simulink model "FCElectricPlant"  (R2025b)
settings: Solver=VariableStepAuto  StartTime=0.0  StopTime=2474  RelTol=1e-3
model workspace (MAT data in the model file):
  Bat : object (value not decoded)
  BattDCDC : object (value not decoded)
  Brk : object (value not decoded)
  Cond : object (value not decoded)
  Cpl : object (value not decoded)
  DH2 = 74
  DH2O = 25
  DO2 = 18
  DRVctrl : object (value not decoded)
  Diff : object (value not decoded)
  Driveshaft : inertia (value not decoded)
  Duct : object (value not decoded)
  ElecThermal : object (value not decoded)
  FCDCDC : object (value not decoded)
  FCctrl : object (value not decoded)
  FTP72 : object (value not decoded)
  FTP75 : object (value not decoded)
  FinArea = 2
  FinDensity = 4
  H2_D = 74
  H2_R = 4124.48151676
  H2_T = [-56.55 -50 -40 -30 -20 -10 -5 -4 -3 -2 -1 0 ... (52 elements, 1x52)]
  H2_h = [2783.66044046 2873.94181646 3012.62601981 3152.22537302 3292.62486344 3433.7213836 3504.50184296 3518.67512521 3532.85394544 3547.03822323 3561.22787913 3575.42283463 ... (52 elements, 1x52)]
  H2_k = [142.834673487 146.602208511 152.236222043 157.732550942 163.09765294 168.338595937 170.914793442 171.426608923 171.937300227 172.446874689 172.955339635 173.462702375 ... (52 elements, 1x52)]
  H2_mu = [7.13280985169 7.28192581803 7.50683010986 7.72860158312 7.94743907375 8.16352107178 8.27057966039 8.29191522386 8.31322574339 8.33451136221 8.35577222214 8.37700846366 ... (52 elements, 1x52)]
  HWFET : object (value not decoded)
  Mot : object (value not decoded)
  N2_R = 296.802103844
  N2_T = [-56.55 -50 -40 -30 -20 -10 -5 -4 -3 -2 -1 0 ... (52 elements, 1x52)]
  N2_h = [224.312019476 231.141016529 241.564116975 251.984329606 262.402210767 272.818266127 278.025759131 279.06722248 280.10867517 281.150117667 282.191550441 283.232973957 ... (52 elements, 1x52)]
  N2_k = [19.6296532607 20.1533289725 20.9436243616 21.7231523445 22.4923063139 23.2514823267 23.6274403303 23.7023472872 23.7771601873 23.8518793809 23.9265052168 24.0010380424 ... (52 elements, 1x52)]
  N2_mu = [13.7948920665 14.1367187352 14.6513506072 15.1575394446 15.6556177861 16.1459023391 16.3882166949 16.4364580271 16.4846261831 16.532721447 16.5807441017 16.6286944287 ... (52 elements, 1x52)]
  NFin = 7680
  O2_D = 18
  O2_R = 259.836612623
  O2_T = [-56.55 -50 -40 -30 -20 -10 -5 -4 -3 -2 -1 0 ... (52 elements, 1x52)]
  O2_h = [196.314045635 202.302438243 211.445560194 220.590899229 229.740231593 238.895348953 243.475641264 244.39194743 245.308340402 246.224821996 247.14139403 248.05805832 ... (52 elements, 1x52)]
  O2_k = [19.6661951881 20.2224765128 21.0645207725 21.898029696 22.7232456338 23.5404090718 23.9460452976 24.0269406553 24.1077592592 24.1885013406 24.2691671302 24.349756858 ... (52 elements, 1x52)]
  O2_mu = [15.7665575307 16.1727626079 16.7849249434 17.3877315055 17.9815180942 18.5666055809 18.8559834763 18.9136105725 18.9711555252 19.0286186248 19.0860001607 19.1433004205 ... (52 elements, 1x52)]
  PTctrl : object (value not decoded)
  Pipe : object (value not decoded)
  Pump : object (value not decoded)
  RH2 = 4124.48291466
  RH2O = 461.523115726
  RH_a = 0.6
  RH_c = 0.6
  RN2 = 296.802204439
  RO2 = 259.836700689
  RelayVariant = 1
  ScenarioIndex = 5
  Sig : Simulink.Signal (value not decoded)
  SimEndTime = 2474
  T_cell = 80
  T_eff_bp = [0 20 40 60 80 100 120 140 160 180 200 220 ... (15 elements, 1x15)]
  T_env = 20
  T_ext = 30
  T_init = 303.15
  Tank : object (value not decoded)
  Tire : object (value not decoded)
  Tvec = [-50 -40 -30 -20 -10 0 10 20 30 40 50 60 ... (41 elements, 1x41)]
  US06 : object (value not decoded)
  UrbanCycle1 : object (value not decoded)
  UrbanCycle2 : object (value not decoded)
  UrbanCycle3 : object (value not decoded)
  UrbanCycle4 : object (value not decoded)
  UrbanCycle5 : object (value not decoded)
  Vehicle : object (value not decoded)
  WOT : object (value not decoded)
  anode_tube_D = 0.01
  cathode_tube_D = 0.05
  comp_mdot_corr_TLU = [0 0 0 0 0 0.2 0.15 0.1 0.05 0 0.4 0.3 ... (15 elements, 5x3)]
  comp_p_ratio_TLU = [1; 1.25; 1.5; 1.75; 2]
  comp_rpm_TLU = [0 1800 3600]
  coolant_num_layers = 20
  coolant_num_passes = 12
  coolant_tube_D = 0.05
  coolant_w_channels = 1
  drive_cycle_power = [0 0 0 0 0 0 0 0 0 0 0 0 ... (1050 elements, 1050x1)]
  drive_cycle_time = [0 3.15544362088e-30 0.0046730644306 0.0046730644306 0.0229169980413 0.0229169980413 0.0411609316521 0.0594048652628 0.0958927324843 0.168868466927 0.308339923682 0.308339923682 ... (1050 elements, 1050x1)]
  efficiency_table = [85 85 85 85 85 85 85 85 85 85 85 85 ... (180 elements, 12x15)]
  env_RH = 0.5
  env_T = 20
  env_p = 0.101325
  env_yO2 = 0.21
  f_fc_auxpower = [551.873653203 546.0853282 528.48462663 513.173595038 503.302975177 502.753456089 515.021163214 542.265022773 584.751680012 640.816461254 707.312051903 780.384247238 ... (869 elements, 79x11)]
  f_fc_currcmd_bpt = [0.209765 5.20060185897 10.1914387179 15.1822755769 20.1731124359 25.1639492949 30.1547861538 35.1456230128 40.1364598718 45.1272967308 50.1181335897 55.1089704487 ... (79 elements, 1x79)]
  f_fc_h2flow = [8.71593619412e-08 2.11208831613e-05 4.21802637945e-05 6.3315607286e-05 8.44733435522e-05 0.000105614873893 0.000126714989157 0.000147760022647 0.000168745833381 0.000189675717181 0.000210558338983 0.000231405772833 ... (869 elements, 79x11)]
  f_fc_heatflow = [-113.508553924 315.682858012 683.83093304 1077.33211881 1492.74924564 1928.28255982 2383.1090309 2856.86201514 3349.28475785 3860.05320307 4388.73420272 4934.82889994 ... (869 elements, 79x11)]
  f_fc_tmpcmd_bpt = [50 55 60 65 70 75 80 85 90 95 100]
  f_fc_voltage = [454.992615106 449.926167951 444.44198715 439.413829244 434.829610174 430.668984057 426.90491616 423.505302786 420.434569606 417.655187333 415.129053553 412.818701247 ... (869 elements, 79x11)]
  hH2 = [2873941.81645 3012626.01981 3152225.37301 3292624.86344 3433721.38359 3575422.83463 3717647.2553 3860321.98734 4003382.88163 4146773.54613 4290444.63593 4434353.18483 ... (41 elements, 1x41)]
  hH2O = [2407979.18389 2426599.35505 2445219.52621 2463839.69737 2482459.86853 2501080.03969 2520041.36444 2538661.5356 2557304.93352 2575974.09714 2594671.5511 2613399.77792 ... (41 elements, 1x41)]
  hN2 = [231141.016491 241564.116943 251984.329578 262402.210743 272818.266107 283232.973942 293646.803464 304060.22922 314473.742203 324887.858166 335303.123505 345720.119022 ... (41 elements, 1x41)]
  hO2 = [202302.438244 211445.560195 220590.89923 229740.231594 238895.348953 248058.05832 257230.174606 266413.508634 275609.852766 284820.965752 294048.557919 303294.277514 ... (41 elements, 1x41)]
  hvH2O = [2837864.0802 2838666.81899 2838713.54467 2838009.25742 2836579.406 2834477.18894 2477187.06302 2453519.25942 2429811.22988 2405977.28679 2381947.12654 2357654.5203 ... (41 elements, 1x41)]
  kH2 = [0.14660211438 0.15223611697 0.157732436203 0.163097529696 0.168338465237 0.173462565161 0.178477161614 0.183389433463 0.188206302164 0.192934369439 0.197579884152 0.202148729169 ... (41 elements, 1x41)]
  kH2O = [0.0133993325489 0.0140727292017 0.0147461258545 0.0154195225073 0.0160929191601 0.0167663158129 0.017416450238 0.0180898468908 0.0187835182831 0.019496836926 0.0202291830642 0.0209799564979 ... (41 elements, 1x41)]
  kN2 = [0.0201533289599 0.0209436243479 0.0217231523299 0.0224923062983 0.0232514823103 0.0240010380251 0.0247413260421 0.0254726839711 0.026195434744 0.0269098870397 0.0276163357829 0.028315062687 ... (41 elements, 1x41)]
  kO2 = [0.0202224764979 0.0210645207571 0.0218980296803 0.0227232456176 0.0235404090551 0.0243497568408 0.0251515209302 0.0259459275017 0.0267331962527 0.0275135401488 0.0282871691008 0.0290542796888 ... (41 elements, 1x41)]
  muH2 = [7.28192631884e-06 7.50683062629e-06 7.72860211493e-06 7.94743962074e-06 8.16352163375e-06 8.37700904042e-06 8.58804741514e-06 8.79676894741e-06 9.00329407235e-06 9.20773285791e-06 9.41018619135e-06 9.61074679906e-06 ... (41 elements, 1x41)]
  muH2O = [7.40754821278e-06 7.71570492949e-06 8.0238616462e-06 8.33201836291e-06 8.64017507962e-06 8.94833179633e-06 9.24231634895e-06 9.55047306566e-06 9.87031914628e-06 1.02003383346e-05 1.05392900589e-05 1.08861429187e-05 ... (41 elements, 1x41)]
  muN2 = [1.41367187228e-05 1.46513505944e-05 1.51575394313e-05 1.56556177724e-05 1.6145902325e-05 1.66286944141e-05 1.71042805521e-05 1.75729330776e-05 1.80349108304e-05 1.84904598363e-05 1.89398139868e-05 1.9383195703e-05 ... (41 elements, 1x41)]
  muO2 = [1.6172762594e-05 1.67849249289e-05 1.73877314906e-05 1.79815180788e-05 1.8566605565e-05 1.9143300404e-05 1.97118951916e-05 2.02726692488e-05 2.08258892185e-05 2.13718096611e-05 2.19106736419e-05 2.24427133044e-05 ... (41 elements, 1x41)]
  pH2O = [0.0039376926592 0.0128411282011 0.0380050105363 0.103238678713 0.259872929049 0.611151401419 1.22819893069 2.33931818334 4.24697083683 7.38493807375 12.3519458375 19.9464343078 ... (41 elements, 1x41)]
  p_a = 0.101325
  p_c = 0.101325
  p_sat = 0.0474144740302
  p_sat_c = 0.0474144740302
  p_sat_e = 0.00233931818334
  radiator_H = 0.5
  radiator_L = 1
  radiator_N_fins = 12000
  radiator_N_tubes = 25
  radiator_W = 0.025
  radiator_air_area_fins = 11.5625
  radiator_air_area_primary = 1.223125
  radiator_cp = 910
  radiator_eta_fin = 0.7
  radiator_fin_spacing = 0.002
  radiator_gap_H = 0.0192708333333
  radiator_rho = 2700
  radiator_t_wall = 0.0001
  radiator_tube_H = 0.0015
  radiator_tube_Leq = 2.5
  stack_D_gdl = 0.07
  stack_alpha = 0.6
  stack_area = 280
  stack_iL = 1.4
  stack_io = 0.0001
  stack_mea_cp = 870
  stack_mea_rho = 1800
  stack_membrane_MW = 1.1
  stack_membrane_rho = 2000
  stack_num_cells = 400
  stack_num_channels = 8
  stack_t_gdl = 250
  stack_t_membrane = 125
  stack_w_channels = 1
  tank_V = 120
  tank_p = 70
  tank_yH2 = 0.9997
  y_H2O_a = 0.280766685597
  y_H2O_c = 0.0138523652603
  y_H2_a = 0.719233314403
  y_N2_a = 0
  y_N2_c = 0.77614763474
  y_O2_c = 0.21
symbols that are objects in the model workspace (value not decoded): Bat, ElecThermal, Mot
libraries: fl_lib x91, nesl_utility x43, autolibpowerinfoutils x9, SimscapeFluids_lib x5, ee_lib x3, slpidlib x2, batteryecm_lib x1, simulink_extras x1, simulink x1
(part 4 of 4)

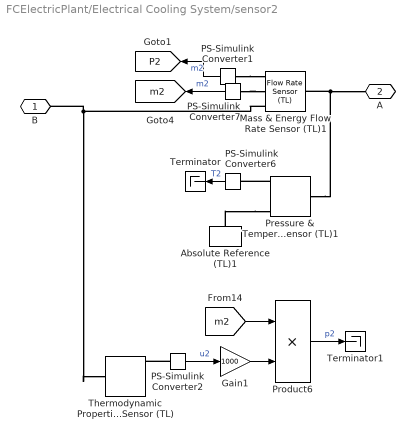
== system FCElectricPlant/Electrical Cooling System/sensor2 ==
  Absolute Reference (TL)1 : fl_lib/Thermal Liquid/Elements/Absolute Reference (TL)
  Gain1 : Gain  Gain=1000
  Mass & Energy Flow Rate Sensor (TL)1 : fl_lib/Thermal Liquid/Sensors/Flow Rate Sensor (TL)  mass_flow_measure=true  volumetric_flow_measure=false  energy_flow_measure=true
      settings: InternalSimscapePortConfiguration="{\"Bottom\":[{\"id\":\"PHI\",\"label\":\"φ\",\"type\":\"output\"}],\"Left\":[{\"id\":\"A\",\"label\":\"A\",\"type\":\"foundation.thermal_liquid.thermal_liquid\"}],\"Right\":[{\"id\":\"B\",\"label\":\"B\",\"type\":\"foundation.thermal_liquid.thermal_liquid\"},{\"id\":\"M\",\"label\":\"M\",\"type\":\"output\"}],\"Top\":[]}"
  PS-Simulink Converter{1..2,6..7} (4 alike) : nesl_utility/PS-Simulink Converter  PhysicalDomain=network_engine_domain  SubClassName=ps_output  LeftPortType=input  RightPortType=output  PseudoPeriodic=off  Frequencies=[]  VectorFormat=inherit  Unit=inherit  AffineConversion=off
  Pressure & Temperature Sensor (TL)1 : fl_lib/Thermal Liquid/Sensors/Pressure & Temperature Sensor (TL)  reference=foundation.enum.MeasurementReference.difference  pressure=true  pressure_spec=foundation.enum.PressureMeasementSpec.Absolute  temperature=true
      settings: InternalSimscapePortConfiguration="{\"Bottom\":[{\"id\":\"T\",\"label\":\"T\",\"type\":\"output\"}],\"Left\":[{\"id\":\"A\",\"label\":\"A\",\"type\":\"foundation.thermal_liquid.thermal_liquid\"}],\"Right\":[{\"id\":\"B\",\"label\":\"B\",\"type\":\"foundation.thermal_liquid.thermal_liquid\"},{\"id\":\"P\",\"label\":\"P\",\"type\":\"output\"}],\"Top\":[]}"
  Product6 : Product
  Terminator : Terminator
  Terminator1 : Terminator
  Thermodynamic Properties Sensor (TL) : fl_lib/Thermal Liquid/Sensors/Thermodynamic Properties Sensor (TL)  internal_energy=true  density=true  specific_heat=true
      settings: InternalSimscapePortConfiguration="{\"Bottom\":[],\"Left\":[{\"id\":\"A\",\"label\":\"A\",\"type\":\"foundation.thermal_liquid.thermal_liquid\"}],\"Right\":[{\"id\":\"U\",\"label\":\"u\",\"type\":\"output\"},{\"id\":\"RHO\",\"label\":\"ρ\",\"type\":\"output\"},{\"id\":\"CP\",\"label\":\"cp\",\"type\":\"output\"}],\"Top\":[]}"
  B : PMIOPort  Side=Left
  A : PMIOPort  Port=2  Side=Right
  tag scope: P2=global, m2=global
  wires:
  PS-Simulink Converter6/1 -> Terminator/1  "T2"
  PS-Simulink Converter7/1 -> [m2]  "m2"
  Product6/1 -> Terminator1/1  "p2"
  Gain1/1 -> Product6/2
  PS-Simulink Converter2/1 -> Gain1/1  "u2"
  [m2] -> Product6/1
  PS-Simulink Converter1/1 -> [P2]  "m2"
  connections:
  Pressure & Temperature Sensor (TL)1/LConn1 -- A/RConn1 -- Mass & Energy Flow Rate Sensor (TL)1/LConn1
  PS-Simulink Converter7/LConn1 -- Mass & Energy Flow Rate Sensor (TL)1/RConn2
  Mass & Energy Flow Rate Sensor (TL)1/RConn1 -- Thermodynamic Properties Sensor (TL)/LConn1 -- B/RConn1
  Pressure & Temperature Sensor (TL)1/RConn3 -- PS-Simulink Converter6/LConn1
  PS-Simulink Converter2/LConn1 -- Thermodynamic Properties Sensor (TL)/RConn1
  Absolute Reference (TL)1/LConn1 -- Pressure & Temperature Sensor (TL)1/RConn1
  PS-Simulink Converter1/LConn1 -- Mass & Energy Flow Rate Sensor (TL)1/RConn3

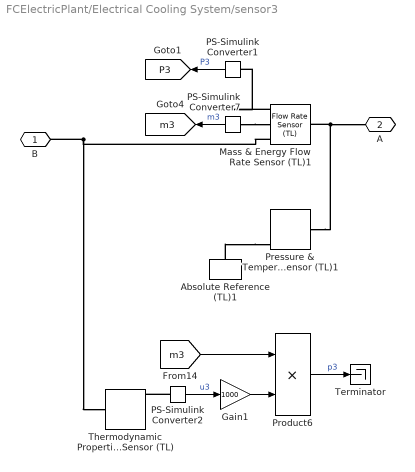
== system FCElectricPlant/Electrical Cooling System/sensor3 ==
  Absolute Reference (TL)1 : fl_lib/Thermal Liquid/Elements/Absolute Reference (TL)
  Gain1 : Gain  Gain=1000
  Mass & Energy Flow Rate Sensor (TL)1 : fl_lib/Thermal Liquid/Sensors/Flow Rate Sensor (TL)  mass_flow_measure=true  volumetric_flow_measure=false  energy_flow_measure=true
      settings: InternalSimscapePortConfiguration="{\"Bottom\":[{\"id\":\"PHI\",\"label\":\"φ\",\"type\":\"output\"}],\"Left\":[{\"id\":\"A\",\"label\":\"A\",\"type\":\"foundation.thermal_liquid.thermal_liquid\"}],\"Right\":[{\"id\":\"B\",\"label\":\"B\",\"type\":\"foundation.thermal_liquid.thermal_liquid\"},{\"id\":\"M\",\"label\":\"M\",\"type\":\"output\"}],\"Top\":[]}"
  PS-Simulink Converter1 : nesl_utility/PS-Simulink Converter  PhysicalDomain=network_engine_domain  SubClassName=ps_output  LeftPortType=input  RightPortType=output  PseudoPeriodic=off  Frequencies=[]  VectorFormat=inherit  Unit=inherit  AffineConversion=off
  PS-Simulink Converter2 : nesl_utility/PS-Simulink Converter  PhysicalDomain=network_engine_domain  SubClassName=ps_output  LeftPortType=input  RightPortType=output  PseudoPeriodic=off  Frequencies=[]  VectorFormat=inherit  Unit=inherit  AffineConversion=off
  PS-Simulink Converter7 : nesl_utility/PS-Simulink Converter  PhysicalDomain=network_engine_domain  SubClassName=ps_output  LeftPortType=input  RightPortType=output  PseudoPeriodic=off  Frequencies=[]  VectorFormat=inherit  Unit=inherit  AffineConversion=off
  Pressure & Temperature Sensor (TL)1 : fl_lib/Thermal Liquid/Sensors/Pressure & Temperature Sensor (TL)  reference=foundation.enum.MeasurementReference.difference  pressure=true  pressure_spec=foundation.enum.PressureMeasementSpec.Absolute  temperature=true
      settings: InternalSimscapePortConfiguration="{\"Bottom\":[{\"id\":\"T\",\"label\":\"T\",\"type\":\"output\"}],\"Left\":[{\"id\":\"A\",\"label\":\"A\",\"type\":\"foundation.thermal_liquid.thermal_liquid\"}],\"Right\":[{\"id\":\"B\",\"label\":\"B\",\"type\":\"foundation.thermal_liquid.thermal_liquid\"},{\"id\":\"P\",\"label\":\"P\",\"type\":\"output\"}],\"Top\":[]}"
  Product6 : Product
  Terminator : Terminator
  Thermodynamic Properties Sensor (TL) : fl_lib/Thermal Liquid/Sensors/Thermodynamic Properties Sensor (TL)  internal_energy=true  density=true  specific_heat=true
      settings: InternalSimscapePortConfiguration="{\"Bottom\":[],\"Left\":[{\"id\":\"A\",\"label\":\"A\",\"type\":\"foundation.thermal_liquid.thermal_liquid\"}],\"Right\":[{\"id\":\"U\",\"label\":\"u\",\"type\":\"output\"},{\"id\":\"RHO\",\"label\":\"ρ\",\"type\":\"output\"},{\"id\":\"CP\",\"label\":\"cp\",\"type\":\"output\"}],\"Top\":[]}"
  B : PMIOPort  Side=Left
  A : PMIOPort  Port=2  Side=Right
  tag scope: P3=global, m3=global
  wires:
  [m3] -> Product6/1
  PS-Simulink Converter2/1 -> Gain1/1  "u3"
  Gain1/1 -> Product6/2
  PS-Simulink Converter7/1 -> [m3]  "m3"
  PS-Simulink Converter1/1 -> [P3]  "P3"
  Product6/1 -> Terminator/1  "p3"
  connections:
  Absolute Reference (TL)1/LConn1 -- Pressure & Temperature Sensor (TL)1/RConn1
  PS-Simulink Converter2/LConn1 -- Thermodynamic Properties Sensor (TL)/RConn1
  B/RConn1 -- Thermodynamic Properties Sensor (TL)/LConn1 -- Mass & Energy Flow Rate Sensor (TL)1/RConn1
  PS-Simulink Converter7/LConn1 -- Mass & Energy Flow Rate Sensor (TL)1/RConn2
  Mass & Energy Flow Rate Sensor (TL)1/LConn1 -- A/RConn1 -- Pressure & Temperature Sensor (TL)1/LConn1
  Mass & Energy Flow Rate Sensor (TL)1/RConn3 -- PS-Simulink Converter1/LConn1

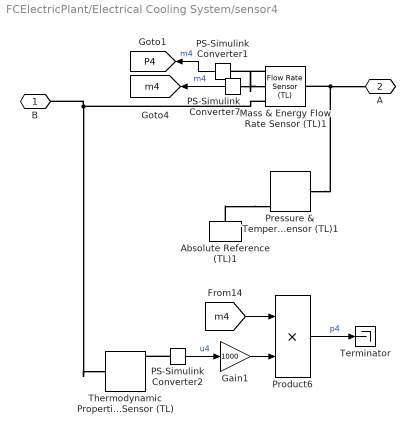
== system FCElectricPlant/Electrical Cooling System/sensor4 ==
  Absolute Reference (TL)1 : fl_lib/Thermal Liquid/Elements/Absolute Reference (TL)
  Gain1 : Gain  Gain=1000
  Mass & Energy Flow Rate Sensor (TL)1 : fl_lib/Thermal Liquid/Sensors/Flow Rate Sensor (TL)  mass_flow_measure=true  volumetric_flow_measure=false  energy_flow_measure=true
      settings: InternalSimscapePortConfiguration="{\"Bottom\":[{\"id\":\"PHI\",\"label\":\"φ\",\"type\":\"output\"}],\"Left\":[{\"id\":\"A\",\"label\":\"A\",\"type\":\"foundation.thermal_liquid.thermal_liquid\"}],\"Right\":[{\"id\":\"B\",\"label\":\"B\",\"type\":\"foundation.thermal_liquid.thermal_liquid\"},{\"id\":\"M\",\"label\":\"M\",\"type\":\"output\"}],\"Top\":[]}"
  PS-Simulink Converter1 : nesl_utility/PS-Simulink Converter  PhysicalDomain=network_engine_domain  SubClassName=ps_output  LeftPortType=input  RightPortType=output  PseudoPeriodic=off  Frequencies=[]  VectorFormat=inherit  Unit=inherit  AffineConversion=off
  PS-Simulink Converter2 : nesl_utility/PS-Simulink Converter  PhysicalDomain=network_engine_domain  SubClassName=ps_output  LeftPortType=input  RightPortType=output  PseudoPeriodic=off  Frequencies=[]  VectorFormat=inherit  Unit=inherit  AffineConversion=off
  PS-Simulink Converter7 : nesl_utility/PS-Simulink Converter  PhysicalDomain=network_engine_domain  SubClassName=ps_output  LeftPortType=input  RightPortType=output  PseudoPeriodic=off  Frequencies=[]  VectorFormat=inherit  Unit=inherit  AffineConversion=off
  Pressure & Temperature Sensor (TL)1 : fl_lib/Thermal Liquid/Sensors/Pressure & Temperature Sensor (TL)  reference=foundation.enum.MeasurementReference.difference  pressure=true  pressure_spec=foundation.enum.PressureMeasementSpec.Absolute  temperature=true
      settings: InternalSimscapePortConfiguration="{\"Bottom\":[{\"id\":\"T\",\"label\":\"T\",\"type\":\"output\"}],\"Left\":[{\"id\":\"A\",\"label\":\"A\",\"type\":\"foundation.thermal_liquid.thermal_liquid\"}],\"Right\":[{\"id\":\"B\",\"label\":\"B\",\"type\":\"foundation.thermal_liquid.thermal_liquid\"},{\"id\":\"P\",\"label\":\"P\",\"type\":\"output\"}],\"Top\":[]}"
  Product6 : Product
  Terminator : Terminator
  Thermodynamic Properties Sensor (TL) : fl_lib/Thermal Liquid/Sensors/Thermodynamic Properties Sensor (TL)  internal_energy=true  density=true  specific_heat=true
      settings: InternalSimscapePortConfiguration="{\"Bottom\":[],\"Left\":[{\"id\":\"A\",\"label\":\"A\",\"type\":\"foundation.thermal_liquid.thermal_liquid\"}],\"Right\":[{\"id\":\"U\",\"label\":\"u\",\"type\":\"output\"},{\"id\":\"RHO\",\"label\":\"ρ\",\"type\":\"output\"},{\"id\":\"CP\",\"label\":\"cp\",\"type\":\"output\"}],\"Top\":[]}"
  B : PMIOPort  Side=Left
  A : PMIOPort  Port=2  Side=Right
  tag scope: P4=global, m4=global
  wires:
  PS-Simulink Converter7/1 -> [m4]  "m4"
  Product6/1 -> Terminator/1  "p4"
  Gain1/1 -> Product6/2
  PS-Simulink Converter2/1 -> Gain1/1  "u4"
  [m4] -> Product6/1
  PS-Simulink Converter1/1 -> [P4]  "m4"
  connections:
  Pressure & Temperature Sensor (TL)1/LConn1 -- A/RConn1 -- Mass & Energy Flow Rate Sensor (TL)1/LConn1
  PS-Simulink Converter7/LConn1 -- Mass & Energy Flow Rate Sensor (TL)1/RConn2
  Mass & Energy Flow Rate Sensor (TL)1/RConn1 -- Thermodynamic Properties Sensor (TL)/LConn1 -- B/RConn1
  PS-Simulink Converter2/LConn1 -- Thermodynamic Properties Sensor (TL)/RConn1
  Absolute Reference (TL)1/LConn1 -- Pressure & Temperature Sensor (TL)1/RConn1
  Mass & Energy Flow Rate Sensor (TL)1/RConn3 -- PS-Simulink Converter1/LConn1

== system FCElectricPlant/Fuel Cell/Converter Control ==
  FCCurrCmd : Inport
  FCCurr : Inport  Port=2
  Add : Sum
  Add1 : Sum  Inputs=-+
  Compare To Constant : simulink/Logic and Bit Operations/Compare To Constant  relop=<=  const=0.01  OutDataTypeStr=boolean  ZeroCross=off
  Constant : Constant  Value=0
  Constant3 : Constant  Value=0
  PID Controller : slpidlib/PID Controller  Controller=PID  Form=Parallel  TimeDomain=Continuous-time  UseExternalTs=off  SampleTime=-1  IntegratorMethod=Forward Euler  FilterMethod=Forward Euler  ControllerParametersSource=internal  P=0.006  I=0.01  UseKiTs=off  D=0  UseExternalDerivativeSource=off  N=100  UseFilter=on  TunerSelectOption=Transfer Function Based (PID Tuner App)  InitialConditionSource=external  InitialConditionForIntegrator=0  InitialConditionForFilter=0  DifferentiatorICPrevScaledInput=0  ExternalReset=falling  TrackingMode=off  Kt=1  LimitOutput=on  SatLimitsSource=internal  UpperSaturationLimit=1  LowerSaturationLimit=-1  LinearizeAsGain=on  AntiWindupMode=none  Kb=1  LimitIntegrator=off  UpperIntegratorSaturationLimit=inf  LowerIntegratorSaturationLimit=-inf  POutMin=[]  POutMax=[]  IOutMin=[]  IOutMax=[]  DOutMin=[]  DOutMax=[]  NOutMin=[]  NOutMax=[]  SumOutMin=[]  SumOutMax=[]  SaturationOutMin=[]  SaturationOutMax=[]  PParamMin=[]  PParamMax=[]  IParamMin=[]  IParamMax=[]  DParamMin=[]  DParamMax=[]  NParamMin=[]  NParamMax=[]  KbParamMin=[]  KbParamMax=[]  KtParamMin=[]  KtParamMax=[]  KbOutMin=[]  KbOutMax=[]  KtOutMin=[]  KtOutMax=[]  IntegratorOutMin=[]  IntegratorOutMax=[]  FilterOutMin=[]  FilterOutMax=[]  SumI1OutMin=[]  SumI1OutMax=[]  SumI2OutMin=[]  SumI2OutMax=[]  SumI3OutMin=[]  SumI3OutMax=[]  SumI4OutMin=[]  SumI4OutMax=[]  SumDOutMin=[]  SumDOutMax=[]  DifferentiatorOutMin=[]  DifferentiatorOutMax=[]  FilterDiffOutCoefMin=[]  FilterDiffOutCoefMax=[]  ReciprocalOutMin=[]  ReciprocalOutMax=[]  SumDenOutMin=[]  SumDenOutMax=[]  SumNumOutMin=[]  SumNumOutMax=[]  DivideOutMin=[]  DivideOutMax=[]  UdiffTsProdOutMin=[]  UdiffTsProdOutMax=[]  NTsProdOutMin=[]  NTsProdOutMax=[]  UintegralTsProdOutMin=[]  UintegralTsProdOutMax=[]  UngainTsProdOutMin=[]  UngainTsProdOutMax=[]  ClampingZeroOutDataTypeStr=Inherit: Inherit via back propagation  ClampingZeroOutMin=[]  ClampingZeroOutMax=[]  FilterDenConstantOutDataTypeStr=Inherit: Inherit via back propagation  FilterDenConstantOutMin=[]  FilterDenConstantOutMax=[]  PCopyOutDataTypeStr=Inherit: Inherit via back propagation  PCopyOutMin=[]  PCopyOutMax=[]  NCopyOutDataTypeStr=Inherit: Inherit via back propagation  NCopyOutMin=[]  NCopyOutMax=[]  IntegratorContinuousStateAttributes=''  IntegratorStateMustResolveToSignalObject=off  IntegratorRTWStateStorageClass=Auto  FilterContinuousStateAttributes=''  FilterStateMustResolveToSignalObject=off  FilterRTWStateStorageClass=Auto  ParallelPVariant=InternalParameters  IdealPVariant=Disabled  IVariant=InternalParameters  DVariant=InternalParameters  IntegratorVariant=Continuous  SatVariant=Enabled  AWVariant=Passthrough  PCopyVariant=Disabled  TRVariant=Disabled  FdbkBlocksVariant=Forward  IdealPFdbkVariant=Disabled  SatFdbkVariant=Disabled  DerivativeFilterVariant=ContFilter  NVariant=InternalParameters  NCopyVariant=Disabled  FilterICVariant=ExternalICs  IntegratorICVariant=ExternalICs  ExternalResetVariant=ExternalReset  TRSumVariant=Passthrough  SumFdbkVariant=Disabled  SumVariant=Sum_PID  TsampFilterVariant=InternalTs  TsampNgainVariant=Passthrough  TsampIntegralVariant=Disabled_SignalSpec  ExternalSaturationOutDataTypeStr=Inherit: Same as second input  DerivativeSourceVariant=ErrorSignal  PreIntVariant=InternalPreInt
  Saturation : Saturate  UpperLimit=1  LowerLimit=0  ZeroCross=off
  Transfer Fcn : TransferFcn  Denominator=[0.001 1]
  u_boost : Outport
  wires:
  Constant3/1 -> Add/2
  PID Controller/1 -> Add/1, Transfer Fcn/1
  FCCurr/1 -> Add1/1
  Add/1 -> Saturation/1
  FCCurrCmd/1 -> Compare To Constant/1, Add1/2
  Add1/1 -> PID Controller/1
  Transfer Fcn/1 -> PID Controller/3
  Constant/1 -> PID Controller/4
  Compare To Constant/1 -> PID Controller/2
  Saturation/1 -> u_boost/1

== system FCElectricPlant/Fuel Cell/Fuel Cell ==
  i_cmd : Inport
  FCTempCmd : Inport  Port=2
  Lookup Table Fuel Cell : Subsystem  VariantControl=LookupTableFuelCell
      settings: PortSchema="{\"entries\":[{\"content\":{\"sides\":[{\"content\":{\"connectorIds\":[]},\"type\":\"ConnectorPlacement.EquallySpacedRectSide\",\"uuid\":\"32248e1c-8adb-4301-a735-652c844f38d9\"},{\"content\":{\"connectorIds\":[],\"side\":\"RIGHT\"},\"type\":\"ConnectorPlacement.EquallySpacedRectSide\",\"uuid\":\"e199895e-2a46-4791-8ec6-c72fbddb281a\"},{\"content\":{\"connectorIds\":[\"In1\",\"In2\"],\"side\":\"TOP\"},\"type\":\"ConnectorPlacement.EquallySpacedRectSide\",\"uuid\":\"d27f5cfc-8d50-4a08-b63d-60966cdd3a3e\"},{\"content\":{\"connectorIds\":[\"Out1\",\"Out2\",\"Out3\",\"Out4\",\"RConn1\",\"RConn2\"],\"side\":\"BOTTOM\"},\"type\":\"ConnectorPlacement.EquallySpacedRectSide\",\"uuid\":\"4de9f516-5cfd-4c93-92a2-161937995774\"}]},\"type\":\"ConnectorPlacement.EquallySpacedConnector\",\"uuid\":\"ebb74780-6fd4-4e24-9636-290cc1e1e603\"}],\"packageUris\":[\"http://schema.mathworks.com/mf0/Connector/R2020b\"],\"version\":\"1.0\"}"
  Simscape Fuel Cell : Subsystem  VariantControl=SimscapeFuelCell  ReferencedSubsystem=SSCFuelCell
  + : PMIOPort  Side=Right
  - : PMIOPort  Port=2  Side=Right
  FCCurr : Outport
  FCVolt : Outport  Port=2
  Pt : Outport  Port=3
  H2Flow : Outport  Port=4

== system FCElectricPlant/Fuel Cell/Thermal1 ==
  Controlled Heat Flow Rate Source : fl_lib/Thermal/Thermal Sources/Controlled Heat Flow Rate Source
  PS Gain : fl_lib/Physical Signals/Functions/PS Gain  gain=0.001 Ohm
  PS Math Function : fl_lib/Physical Signals/Functions/PS Math Function  fcn_choice=foundation.enum.math_function.square  v=1
  Thermal Mass : fl_lib/Thermal/Thermal Elements/Thermal Mass  mass_type=foundation.enum.constant_variable.constant  mass=500 kg  sp_heat=447 J/kg/K  mass_min=1e-6 kg  num_ports=foundation.enum.numPorts2.one  m_specify=off  m_priority=High  m=1 kg  m_nominal_specify=off  m_nominal_value=1  m_nominal_unit=kg  T_specify=off  T_priority=High  T=300 K  T_nominal_specify=off  T_nominal_value=1  T_nominal_unit=K  Q_specify=off  Q_priority=None  Q=0 W  Q_nominal_specify=off  Q_nominal_value=1  Q_nominal_unit=W
  Thermal Reference2 : fl_lib/Thermal/Thermal Elements/Thermal Reference
  H : PMIOPort  Side=Right
  i : PMIOPort  Port=2  Side=Left
  connections:
  H/RConn1 -- Controlled Heat Flow Rate Source/LConn1 -- Thermal Mass/LConn1
  i/RConn1 -- PS Math Function/LConn1
  Thermal Reference2/LConn1 -- Controlled Heat Flow Rate Source/RConn2
  PS Math Function/RConn1 -- PS Gain/LConn1
  Controlled Heat Flow Rate Source/RConn1 -- PS Gain/RConn1

== system FCElectricPlant/Motor/Elec Sensor ==
  Current Sensor2 : fl_lib/Electrical/Electrical Sensors/Current Sensor
  Electrical Reference : fl_lib/Electrical/Electrical Elements/Electrical Reference
  PS-Simulink Converter : nesl_utility/PS-Simulink Converter  PhysicalDomain=network_engine_domain  SubClassName=ps_output  LeftPortType=input  RightPortType=output  PseudoPeriodic=off  Frequencies=[]  VectorFormat=1-D array  Unit=inherit  AffineConversion=off
  PS-Simulink Converter4 : nesl_utility/PS-Simulink Converter  PhysicalDomain=network_engine_domain  SubClassName=ps_output  LeftPortType=input  RightPortType=output  PseudoPeriodic=off  Frequencies=[]  VectorFormat=1-D array  Unit=1  AffineConversion=off
  Product2 : Product
  Terminator : Terminator
  Voltage Sensor : fl_lib/Electrical/Electrical Sensors/Voltage Sensor
  + : PMIOPort  Side=Left
  - : PMIOPort  Port=2  Side=Right
  wires:
  PS-Simulink Converter4/1 -> Product2/2  "MotCurr"
  Product2/1 -> Terminator/1  "MotPwrElec"
  PS-Simulink Converter/1 -> Product2/1  "MotV"
  connections:
  Current Sensor2/RConn1 -- PS-Simulink Converter4/LConn1
  Current Sensor2/RConn2 -- -/RConn1
  +/RConn1 -- Voltage Sensor/LConn1 -- Current Sensor2/LConn1
  Electrical Reference/LConn1 -- Voltage Sensor/RConn2
  PS-Simulink Converter/LConn1 -- Voltage Sensor/RConn1

== system FCElectricPlant/Motor/Simulink Interface ==
  MotSpd : Inport
  Ideal Angular Velocity Source1 : fl_lib/Mechanical/Mechanical Sources/Ideal Angular Velocity Source
  Ideal Torque Sensor1 : fl_lib/Mechanical/Mechanical Sensors/Ideal Torque Sensor
  Ideal Torque Sensor2 : fl_lib/Mechanical/Mechanical Sensors/Ideal Torque Sensor
  Motor Coupling Dynamics1 : TransferFcn  Denominator=[0.001 1]
  PS-Simulink Converter2 : nesl_utility/PS-Simulink Converter  PhysicalDomain=network_engine_domain  SubClassName=ps_output  LeftPortType=input  RightPortType=output  PseudoPeriodic=off  Frequencies=[]  VectorFormat=1-D array  Unit=1  AffineConversion=off
  Product1 : Product
  Simulink-PS Converter4 : nesl_utility/Simulink-PS Converter  PhysicalDomain=network_engine_domain  SubClassName=ps_input  LeftPortType=input  RightPortType=output  PseudoPeriodic=off  Frequencies=[]  NoiseDistribution=none  NoiseParameters=[]  Unit=rad/s  AffineConversion=off  FilteringAndDerivatives=filter  SimscapeFilterOrder=1  InputFilterTimeConstant=0.001  UdotUserProvided=0
  Terminator : Terminator
  Transfer Fcn2 : TransferFcn  Denominator=[0.001 1]
  C : PMIOPort  Side=Left
  R : PMIOPort  Port=2  Side=Left
  MotTrq : Outport
  wires:
  Motor Coupling Dynamics1/1 -> MotTrq/1  "MotTrq"
  MotSpd/1 -> Transfer Fcn2/1
  PS-Simulink Converter2/1 -> Product1/1, Motor Coupling Dynamics1/1
  Transfer Fcn2/1 -> Product1/2, Simulink-PS Converter4/1
  Product1/1 -> Terminator/1  "MotPwrMech"
  connections:
  Ideal Torque Sensor2/RConn2 -- PS-Simulink Converter2/LConn1
  Ideal Angular Velocity Source1/LConn1 -- Ideal Torque Sensor1/RConn1
  Simulink-PS Converter4/RConn1 -- Ideal Angular Velocity Source1/RConn1
  Ideal Torque Sensor2/RConn1 -- Ideal Torque Sensor1/LConn1
  Ideal Angular Velocity Source1/RConn2 -- C/RConn1
  R/RConn1 -- Ideal Torque Sensor2/LConn1

== system FCElectricPlant/Fuel Cell/Fuel Cell/Lookup Table Fuel Cell ==
  i_cmd : Inport
  FCTempCmd : Inport  Port=2
  Mapped Fuel Cell : Subsystem  mask{f_fc_currcmd_bpt=f_fc_currcmd_bpt, f_fc_tmpcmd_bpt=f_fc_tmpcmd_bpt, f_fc_voltage=f_fc_voltage, f_fc_heatflow=f_fc_heatflow, f_fc_auxpower=f_fc_auxpower, f_fc_h2flow=f_fc_h2flow, CalFuelCellMapData=0, aMode=1}
      mask prompts: f_fc_currcmd_bpt "autoblks:autoblkMappedFuelCellMask:blkPrm_f_fc_currcmd_bpt"; f_fc_tmpcmd_bpt "autoblks:autoblkMappedFuelCellMask:blkPrm_f_fc_tmpcmd_bpt"; f_fc_voltage "autoblks:autoblkMappedFuelCellMask:blkPrm_f_fc_voltage"; f_fc_heatflow "autoblks:autoblkMappedFuelCellMask:blkPrm_f_fc_heatflow"; f_fc_auxpower "autoblks:autoblkMappedFuelCellMask:blkPrm_f_fc_auxpower"; f_fc_h2flow "autoblks:autoblkMappedFuelCellMask:blkPrm_f_fc_h2flow"
      mask DialogControl DescGroupVar Prompt: Mapped Fuel Cell
      mask DialogControl DescTextVar Prompt: autoblks:autoblkMappedFuelCellMask:blkDesc
      mask DialogControl f_fc_currcmd_bpt Prompt: Commanded current, f_fc_currcmd_bpt [A]:
      mask DialogControl f_fc_tmpcmd_bpt Prompt: Commanded temperature, f_fc_tmpcmd_bpt [C]:
      mask DialogControl f_fc_voltage Prompt: Voltage map, f_fc_voltage [V]:
      mask DialogControl f_fc_heatflow Prompt: Heat flow map, f_fc_heatflow [w]:
      mask DialogControl f_fc_auxpower Prompt: Auxiliary power, f_fc_auxpower [w]:
      mask DialogControl f_fc_h2flow Prompt: Hydrogen mass flow rate, f_fc_h2flow [kg/s]:
  + : PMIOPort  Side=Right
  - : PMIOPort  Port=2  Side=Right
  FCCurr : Outport
  FCVolt : Outport  Port=2
  Pt : Outport  Port=3
  H2Flow : Outport  Port=4
  wires:
  i_cmd/1 -> Mapped Fuel Cell/1(i_cmd)
  FCTempCmd/1 -> Mapped Fuel Cell/2(FCTempCmd)
  Mapped Fuel Cell/1(FCCurr) -> FCCurr/1
  Mapped Fuel Cell/2(FCVolt) -> FCVolt/1
  Mapped Fuel Cell/3(AuxPower) -> Pt/1
  Mapped Fuel Cell/4(H2Flow) -> H2Flow/1
  connections:
  Mapped Fuel Cell/RConn1 -- +/RConn1
  Mapped Fuel Cell/RConn2 -- -/RConn1

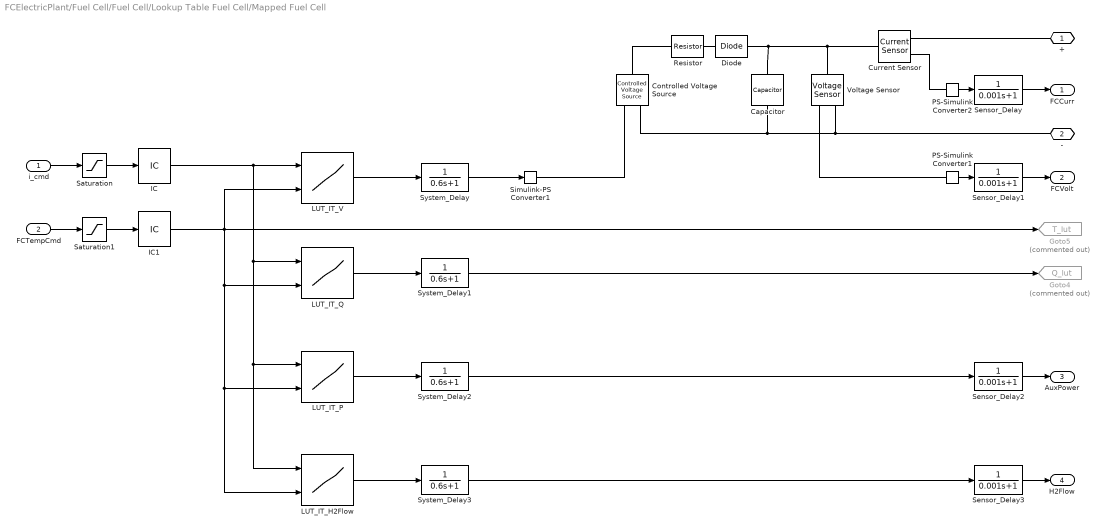
== system FCElectricPlant/Fuel Cell/Fuel Cell/Lookup Table Fuel Cell/Mapped Fuel Cell ==
  i_cmd : Inport
  FCTempCmd : Inport  Port=2
  Capacitor : fl_lib/Electrical/Electrical Elements/Capacitor  c=1e-6 F  r=1e-6 Ohm  g=0 1/Ohm  i_specify=off  i_priority=None  i=0 A  i_nominal_specify=off  i_nominal_value=1  i_nominal_unit=A  v_specify=off  v_priority=None  v=0 V  v_nominal_specify=off  v_nominal_value=1  v_nominal_unit=V  vc_specify=on  vc_priority=High  vc=f_fc_voltage(1) V  vc_nominal_specify=off  vc_nominal_value=1  vc_nominal_unit=V
  Controlled Voltage Source : fl_lib/Electrical/Electrical Sources/Controlled Voltage Source
  Current Sensor : fl_lib/Electrical/Electrical Sensors/Current Sensor
  Diode : fl_lib/Electrical/Electrical Elements/Diode  Vf=0.6 V  Ron=0.3 Ohm  Goff=1e-8 1/Ohm  i_specify=off  i_priority=None  i=0 A  i_nominal_specify=off  i_nominal_value=1  i_nominal_unit=A  v_specify=off  v_priority=None  v=0 V  v_nominal_specify=off  v_nominal_value=1  v_nominal_unit=V
  Goto4 : Goto  Commented=on  GotoTag=Q_lut  TagVisibility=global
  Goto5 : Goto  Commented=on  GotoTag=T_lut  TagVisibility=global
  IC : InitialCondition  Value=f_fc_currcmd_bpt(1)
  IC1 : InitialCondition  Value=f_fc_tmpcmd_bpt(1)
  LUT_IT_H2Flow : Lookup_n-D  BreakpointsForDimension1=f_fc_currcmd_bpt  BreakpointsForDimension2=f_fc_tmpcmd_bpt  Table=f_fc_h2flow  InternalRulePriority=Speed  RndMeth=Simplest
      settings: InputPortMap=u0,u1
  LUT_IT_P : Lookup_n-D  BreakpointsForDimension1=f_fc_currcmd_bpt  BreakpointsForDimension2=f_fc_tmpcmd_bpt  Table=f_fc_auxpower  InternalRulePriority=Speed  RndMeth=Simplest
      settings: InputPortMap=u0,u1
  LUT_IT_Q : Lookup_n-D  BreakpointsForDimension1=f_fc_currcmd_bpt  BreakpointsForDimension2=f_fc_tmpcmd_bpt  Table=f_fc_heatflow  InternalRulePriority=Speed  RndMeth=Simplest
      settings: InputPortMap=u0,u1
  LUT_IT_V : Lookup_n-D  BreakpointsForDimension1=f_fc_currcmd_bpt  BreakpointsForDimension2=f_fc_tmpcmd_bpt  Table=f_fc_voltage  InternalRulePriority=Speed  RndMeth=Simplest
      settings: InputPortMap=u0,u1
  PS-Simulink Converter1 : nesl_utility/PS-Simulink Converter  PhysicalDomain=network_engine_domain  SubClassName=ps_output  LeftPortType=input  RightPortType=output  PseudoPeriodic=off  Frequencies=[]  VectorFormat=1-D array  Unit=inherit  AffineConversion=off
  PS-Simulink Converter2 : nesl_utility/PS-Simulink Converter  PhysicalDomain=network_engine_domain  SubClassName=ps_output  LeftPortType=input  RightPortType=output  PseudoPeriodic=off  Frequencies=[]  VectorFormat=1-D array  Unit=1  AffineConversion=off
  Resistor : fl_lib/Electrical/Electrical Elements/Resistor  R=1e-3 Ohm  i_specify=off  i_priority=None  i=0 A  i_nominal_specify=off  i_nominal_value=1  i_nominal_unit=A  v_specify=off  v_priority=None  v=0 V  v_nominal_specify=off  v_nominal_value=1  v_nominal_unit=V
  Saturation : Saturate  UpperLimit=max(f_fc_currcmd_bpt)  LowerLimit=0
  Saturation1 : Saturate  UpperLimit=max(f_fc_tmpcmd_bpt)  LowerLimit=0
  Sensor_Delay{,1..3} (4 alike) : TransferFcn  Denominator=[0.001 1]
  Simulink-PS Converter1 : nesl_utility/Simulink-PS Converter  PhysicalDomain=network_engine_domain  SubClassName=ps_input  LeftPortType=input  RightPortType=output  PseudoPeriodic=off  Frequencies=[]  NoiseDistribution=none  NoiseParameters=[]  Unit=V  AffineConversion=off  FilteringAndDerivatives=provide  SimscapeFilterOrder=1  InputFilterTimeConstant=0.001  UdotUserProvided=0
  System_Delay{,1..3} (4 alike) : TransferFcn  Denominator=[0.6 1]
  Voltage Sensor : fl_lib/Electrical/Electrical Sensors/Voltage Sensor
  + : PMIOPort  Side=Right
  - : PMIOPort  Port=2  Side=Right
  FCCurr : Outport
  FCVolt : Outport  Port=2
  AuxPower : Outport  Port=3
  H2Flow : Outport  Port=4
  wires:
  PS-Simulink Converter1/1 -> Sensor_Delay1/1
  System_Delay1/1 -> Goto4/1
  Sensor_Delay1/1 -> FCVolt/1
  Sensor_Delay/1 -> FCCurr/1
  PS-Simulink Converter2/1 -> Sensor_Delay/1
  IC/1 -> LUT_IT_H2Flow/1, LUT_IT_P/1, LUT_IT_Q/1, LUT_IT_V/1
  Saturation/1 -> IC/1
  i_cmd/1 -> Saturation/1
  Saturation1/1 -> IC1/1
  FCTempCmd/1 -> Saturation1/1
  IC1/1 -> LUT_IT_V/2, Goto5/1, LUT_IT_H2Flow/2, LUT_IT_P/2, LUT_IT_Q/2
  System_Delay/1 -> Simulink-PS Converter1/1
  LUT_IT_V/1 -> System_Delay/1
  LUT_IT_Q/1 -> System_Delay1/1
  System_Delay2/1 -> Sensor_Delay2/1
  LUT_IT_P/1 -> System_Delay2/1
  System_Delay3/1 -> Sensor_Delay3/1
  LUT_IT_H2Flow/1 -> System_Delay3/1
  Sensor_Delay2/1 -> AuxPower/1
  Sensor_Delay3/1 -> H2Flow/1
  connections:
  Simulink-PS Converter1/RConn1 -- Controlled Voltage Source/RConn1
  PS-Simulink Converter2/LConn1 -- Current Sensor/RConn1
  Controlled Voltage Source/LConn1 -- Resistor/LConn1
  +/RConn1 -- Current Sensor/RConn2
  Controlled Voltage Source/RConn2 -- Capacitor/RConn1 -- Voltage Sensor/RConn2 -- -/RConn1
  Resistor/RConn1 -- Diode/LConn1
  Diode/RConn1 -- Capacitor/LConn1 -- Voltage Sensor/LConn1 -- Current Sensor/LConn1
  PS-Simulink Converter1/LConn1 -- Voltage Sensor/RConn1
